simulink model "bez_aproksimacije"  (Simulink 6.0)
settings: Solver=ode3  StartTime=0.0  StopTime=20  FixedStep=0.001  RelTol=1e-3
values from neighbouring files (symbols this model uses):
  a = input('Unesi vrijednost a:' )    [Kod.m]
  alfa0 = input('Unesi pocetnu vrijednost ugla alfa:' )    [Kod.m]
  beta0 = input('Unesi pocetnu vrijednost ugla beta:')    [Kod.m]
  g = 9.80665    [Kod.m]
  gama0 = input('Unesi pocetnu vrijednost ugla gama:')    [Kod.m]
  k = input('Unesi krutost opruge k:' )    [Kod.m]
  m = input('Unesi masu tijela:')    [Kod.m]
settings Model: LastModifiedBy=Administrator

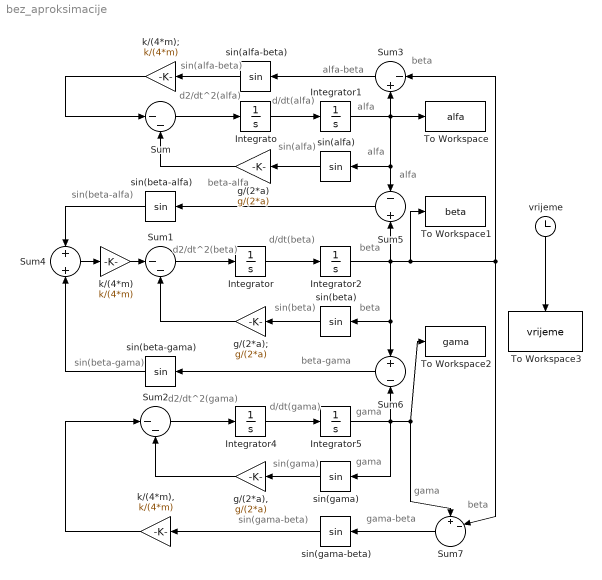
== system bez_aproksimacije ==
  note: d2/dt^2(alfa)
  note: d/dt(alfa)
  note: alfa
  note: d2/dt^2(beta)
  note: d2/dt^2(gama)
  note: d/dt(beta)
  note: gama
  note: gama
  note: beta
  note: alfa
  note: beta
  note: d/dt(gama)
  note: beta
  note: gama-beta
  note: sin(alfa)
  note: alfa-beta
  note: sin(alfa-beta)
  note: beta-alfa
  note: sin(beta-alfa)
  note: beta-gama
  note: sin(beta-gama)
  note: beta
  note: sin(gama-beta)
  note: sin(gama)
  note: sin(beta)
  note: gama
  note: alfa
  Integrato : Integrator
  Integrator : Integrator
  Integrator1 : Integrator  InitialCondition=alfa0
  Integrator2 : Integrator  InitialCondition=beta0
  Integrator4 : Integrator
  Integrator5 : Integrator  InitialCondition=gama0
  Sum : Sum  Inputs=|--  SampleTime=0.001
  Sum1 : Sum  Inputs=|--
  Sum2 : Sum  Inputs=|--
  Sum3 : Sum  Orientation=left  Inputs=|-+
  Sum4 : Sum
  Sum5 : Sum  Orientation=left  Inputs=-|+
  Sum6 : Sum  Orientation=left  Inputs=+|-
  Sum7 : Sum  Orientation=left  Inputs=+-||
  To Workspace : ToWorkspace  VariableName=alfa  SampleTime=-1  SaveFormat=Array
  To Workspace1 : ToWorkspace  VariableName=beta  SampleTime=-1  SaveFormat=Array
  To Workspace2 : ToWorkspace  VariableName=gama  SampleTime=-1  SaveFormat=Array
  To Workspace3 : ToWorkspace  VariableName=vrijeme  SampleTime=-1  SaveFormat=Array
      settings: Orientation=down
  g/(2*a) : Gain  Orientation=left  Gain=g/(2*a)
  g/(2*a), : Gain  Orientation=left  Gain=g/(2*a)
  g/(2*a); : Gain  Orientation=left  Gain=g/(2*a)
  k/(4*m) : Gain  Gain=k/(4*m)
  k/(4*m), : Gain  Orientation=left  Gain=k/(4*m)
  k/(4*m); : Gain  Orientation=left  Gain=k/(4*m)  SampleTime=0.001
  sin(alfa) : Trigonometry  Orientation=left  SampleTime=0.001
  sin(alfa-beta) : Trigonometry  Orientation=left
  sin(beta) : Trigonometry  Orientation=left
  sin(beta-alfa) : Trigonometry  Orientation=left
  sin(beta-gama) : Trigonometry  Orientation=left
  sin(gama) : Trigonometry  Orientation=left
  sin(gama-beta) : Trigonometry  Orientation=left
  vrijeme : Clock
      settings: Orientation=down  Decimation=10
  wires:
  vrijeme/1 -> To Workspace3/1
  g/(2*a),/1 -> Sum2/2
  Integrator5/1 -> sin(gama)/1, To Workspace2/1, Sum7/1, Sum6/2
  Sum2/1 -> Integrator4/1
  Integrator4/1 -> Integrator5/1
  k/(4*m)/1 -> Sum1/1
  g/(2*a);/1 -> Sum1/2
  Integrator2/1 -> To Workspace1/1, Sum3/1, Sum7/2, Sum5/2, sin(beta)/1, Sum6/1
  Sum1/1 -> Integrator/1
  Integrator/1 -> Integrator2/1
  Sum/1 -> Integrato/1
  g/(2*a)/1 -> Sum/2
  Integrator1/1 -> To Workspace/1, Sum3/2, sin(alfa)/1, Sum5/1
  Integrato/1 -> Integrator1/1
  sin(alfa)/1 -> g/(2*a)/1
  sin(alfa-beta)/1 -> k/(4*m);/1
  k/(4*m);/1 -> Sum/1
  Sum3/1 -> sin(alfa-beta)/1
  sin(beta)/1 -> g/(2*a);/1
  Sum4/1 -> k/(4*m)/1
  Sum5/1 -> sin(beta-alfa)/1
  sin(beta-alfa)/1 -> Sum4/1
  Sum6/1 -> sin(beta-gama)/1
  sin(beta-gama)/1 -> Sum4/2
  sin(gama)/1 -> g/(2*a),/1
  Sum7/1 -> sin(gama-beta)/1
  sin(gama-beta)/1 -> k/(4*m),/1
  k/(4*m),/1 -> Sum2/1
